simulink model "inhneutest"  (Simulink 7.6)
settings: Solver=ode45  StartTime=0.0  StopTime=500  RelTol=1e-3
values from neighbouring files (symbols this model uses):
  beta = 0.05    [excneuroninit.m]
  sigslopef = 1    [excneuroninit.m]
  sigslopei = 3    [excneuroninit.m]
  tau_s = 5    [excneuroninit.m]
libraries: simulink x3
settings Model: Creator=root  LastModifiedBy=root

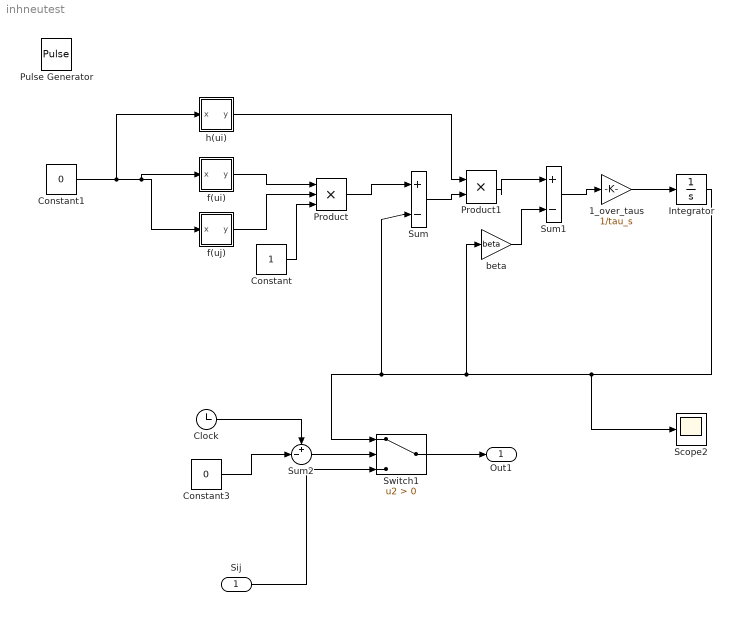
== system inhneutest ==
  Sij : Inport
  1_over_taus : Gain  Gain=1/tau_s
  Clock : Clock
      settings: Decimation=10
  Constant : Constant
  Constant1 : Constant  Value=0
  Constant3 : Constant  Value=0
  Integrator : Integrator
  Product : Product  Inputs=3  RndMeth=Zero
  Product1 : Product  RndMeth=Zero
  Pulse Generator : DiscretePulseGenerator  PulseType=Time based  Amplitude=2  Period=1  PulseWidth=50
  Scope2 : Scope
  Sum : Sum  Inputs=|+-
  Sum1 : Sum  Inputs=|+-
  Sum2 : Sum  Inputs=+-|
  Switch1 : Switch  Criteria=u2 > Threshold
  beta : Gain  Gain=beta
  f(ui) : Subsystem  TreatAsAtomicUnit=on  mask{slope=sigslopef, offset=6}
      mask help: Created by Han, Cheol
      mask Display: plot([10 15 20 25 30 35 40 45 50], [0 0.01 0.1 0.2 0.5 0.8 0.9 0.99 1])
  f(uj) : Subsystem  TreatAsAtomicUnit=on  mask{slope=sigslopef, offset=6}
      mask help: Created by Han, Cheol
      mask Display: plot([10 15 20 25 30 35 40 45 50], [0 0.01 0.1 0.2 0.5 0.8 0.9 0.99 1])
  h(ui) : Subsystem  TreatAsAtomicUnit=on  mask{slope=sigslopei, offset=6}
      mask help: Created by Han, Cheol
      mask Display: plot([10 15 20 25 30 35 40 45 50], [0 0.01 0.1 0.2 0.5 0.8 0.9 0.99 1])
  Out1 : Outport
  wires:
  Constant1/1 -> h(ui)/1(x), f(uj)/1(x), f(ui)/1(x)
  f(ui)/1(y) -> Product/1
  f(uj)/1(y) -> Product/2
  Constant/1 -> Product/3
  Product/1 -> Sum/1
  Sum/1 -> Product1/2
  h(ui)/1(y) -> Product1/1
  Product1/1 -> Sum1/1
  beta/1 -> Sum1/2
  Sum1/1 -> 1_over_taus/1
  1_over_taus/1 -> Integrator/1
  Integrator/1 -> Scope2/1, Switch1/1, Sum/2, beta/1
  Sum2/1 -> Switch1/2
  Clock/1 -> Sum2/1
  Constant3/1 -> Sum2/2
  Switch1/1 -> Out1/1
  Sij/1 -> Switch1/3

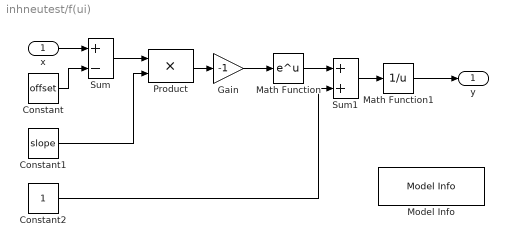
== system inhneutest/f(ui) ==
  x : Inport
  Constant : Constant  Value=offset
  Constant1 : Constant  Value=slope
  Constant2 : Constant
  Gain : Gain  Gain=-1  SaturateOnIntegerOverflow=on  OutDataTypeStr=Inherit: Same as input  ParamDataTypeStr=Inherit: Same as input
  Math Function : Math  SaturateOnIntegerOverflow=on
  Math Function1 : Math  Operator=reciprocal  SaturateOnIntegerOverflow=on
  Model Info : simulink/Model-Wide Utilities/Model Info  SystemSampleTime=-1  InitialBlockCM=None  BlockCM=None  Frame=on  DisplayStringWithTags=|  HorizontalTextAlignment=Center  LeftAlignmentValue=0.5  SourceBlockDiagram=untitled  TagMaxNumber=20
      | Model Info
      | %<Creator> Han, Cheol
  Product : Product  SaturateOnIntegerOverflow=on  OutDataTypeStr=Inherit: Same as first input
  Sum : Sum  Inputs=+-  SaturateOnIntegerOverflow=on
  Sum1 : Sum  SaturateOnIntegerOverflow=on
  y : Outport  InitialOutput=0
  wires:
  x/1 -> Sum/1
  Constant/1 -> Sum/2
  Sum/1 -> Product/1
  Constant1/1 -> Product/2
  Product/1 -> Gain/1
  Gain/1 -> Math Function/1
  Math Function/1 -> Sum1/1
  Constant2/1 -> Sum1/2
  Sum1/1 -> Math Function1/1
  Math Function1/1 -> y/1

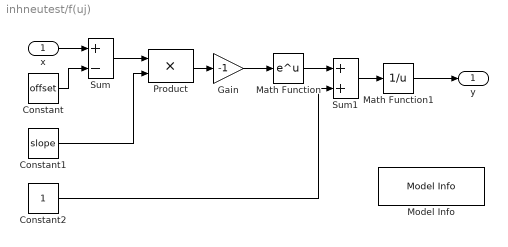
== system inhneutest/f(uj) ==
  x : Inport
  Constant : Constant  Value=offset
  Constant1 : Constant  Value=slope
  Constant2 : Constant
  Gain : Gain  Gain=-1  SaturateOnIntegerOverflow=on  OutDataTypeStr=Inherit: Same as input  ParamDataTypeStr=Inherit: Same as input
  Math Function : Math  SaturateOnIntegerOverflow=on
  Math Function1 : Math  Operator=reciprocal  SaturateOnIntegerOverflow=on
  Model Info : simulink/Model-Wide Utilities/Model Info  SystemSampleTime=-1  InitialBlockCM=None  BlockCM=None  Frame=on  DisplayStringWithTags=|  HorizontalTextAlignment=Center  LeftAlignmentValue=0.5  SourceBlockDiagram=untitled  TagMaxNumber=20
      | Model Info
      | %<Creator> Han, Cheol
  Product : Product  SaturateOnIntegerOverflow=on  OutDataTypeStr=Inherit: Same as first input
  Sum : Sum  Inputs=+-  SaturateOnIntegerOverflow=on
  Sum1 : Sum  SaturateOnIntegerOverflow=on
  y : Outport  InitialOutput=0
  wires:
  x/1 -> Sum/1
  Constant/1 -> Sum/2
  Sum/1 -> Product/1
  Constant1/1 -> Product/2
  Product/1 -> Gain/1
  Gain/1 -> Math Function/1
  Math Function/1 -> Sum1/1
  Constant2/1 -> Sum1/2
  Sum1/1 -> Math Function1/1
  Math Function1/1 -> y/1

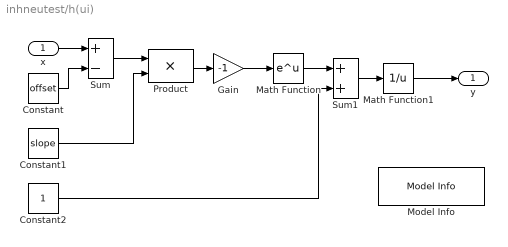
== system inhneutest/h(ui) ==
  x : Inport
  Constant : Constant  Value=offset
  Constant1 : Constant  Value=slope
  Constant2 : Constant
  Gain : Gain  Gain=-1  SaturateOnIntegerOverflow=on  OutDataTypeStr=Inherit: Same as input  ParamDataTypeStr=Inherit: Same as input
  Math Function : Math  SaturateOnIntegerOverflow=on
  Math Function1 : Math  Operator=reciprocal  SaturateOnIntegerOverflow=on
  Model Info : simulink/Model-Wide Utilities/Model Info  SystemSampleTime=-1  InitialBlockCM=None  BlockCM=None  Frame=on  DisplayStringWithTags=|  HorizontalTextAlignment=Center  LeftAlignmentValue=0.5  SourceBlockDiagram=untitled  TagMaxNumber=20
      | Model Info
      | %<Creator> Han, Cheol
  Product : Product  SaturateOnIntegerOverflow=on  OutDataTypeStr=Inherit: Same as first input
  Sum : Sum  Inputs=+-  SaturateOnIntegerOverflow=on
  Sum1 : Sum  SaturateOnIntegerOverflow=on
  y : Outport  InitialOutput=0
  wires:
  x/1 -> Sum/1
  Constant/1 -> Sum/2
  Sum/1 -> Product/1
  Constant1/1 -> Product/2
  Product/1 -> Gain/1
  Gain/1 -> Math Function/1
  Math Function/1 -> Sum1/1
  Constant2/1 -> Sum1/2
  Sum1/1 -> Math Function1/1
  Math Function1/1 -> y/1
